simulink model "lazo_de_torque"  (R2023b)
settings: Solver=VariableStepAuto  StartTime=0.0  StopTime=10.0  RelTol=1e-3
values from neighbouring files (symbols this model uses):
  b_eq = b_m + b_l/(r^2)    (= 2.19444444444e-05)    [constantes.m]    (also in test_polos_PID.m = b_m + b_l_nominal/(r^2))
  k_l = g*(m*l_cm + m_l*l_l)    (= 2.4516625)    [constantes.m]
  lambda_m = 0.016    [constantes.m]
  Ld = 6.6e-3    (= 0.0066)    [constantes.m]
  Lq = 5.8e-3    (= 0.0058)    [constantes.m]
  P_p = 3    [constantes.m]
  r = 120    [constantes.m]
settings Model: Creator=rodri  LastModifiedBy=Nahuel

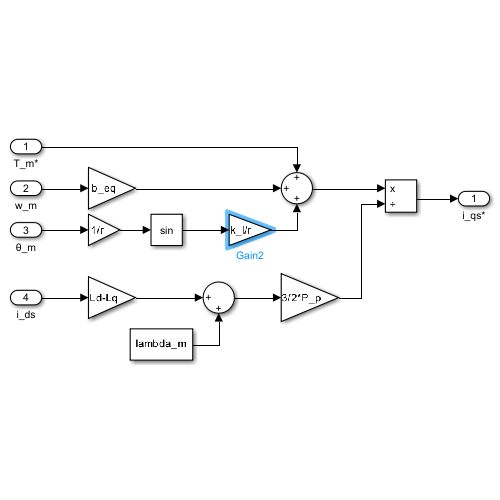
[thumbnail: Simulink's stored preview of the top-level diagram]
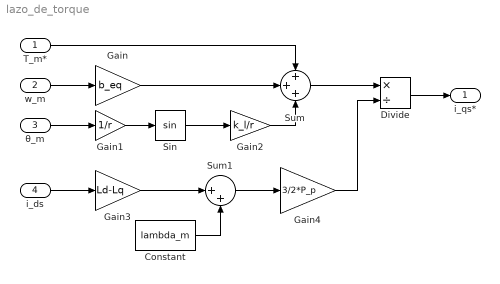
== system lazo_de_torque ==
  T_m* : Inport
  w_m : Inport  Port=2
  θ_m : Inport  Port=3
  i_ds : Inport  Port=4
  Constant : Constant  Value=lambda_m
  Divide : Product  Inputs=*/
  Gain : Gain  Gain=b_eq
  Gain1 : Gain  Gain=1/r
  Gain2 : Gain  Gain=k_l/r
  Gain3 : Gain  Gain=Ld-Lq
  Gain4 : Gain  Gain=3/2*P_p
  Sin : Trigonometry
  Sum : Sum  Inputs=+++
  Sum1 : Sum  Inputs=|++
  i_qs* : Outport
  wires:
  w_m/1 -> Gain/1
  Gain/1 -> Sum/2
  T_m*/1 -> Sum/1
  θ_m/1 -> Gain1/1
  Gain1/1 -> Sin/1
  Sin/1 -> Gain2/1
  Gain2/1 -> Sum/3
  i_ds/1 -> Gain3/1
  Constant/1 -> Sum1/2
  Sum1/1 -> Gain4/1
  Sum/1 -> Divide/1
  Gain4/1 -> Divide/2
  Divide/1 -> i_qs*/1
  Gain3/1 -> Sum1/1
